simulink model "robot_arm"  (Simulink 7.2)
settings: Solver=ode45  StartTime=0.0  StopTime=inf  RelTol=1e-3
libraries: mblibv1 x31, simulink x4, vrlib x1
settings Model: Creator=eniso  LastModifiedBy=houssein01
settings OptimizationCC: InitFltsAndDblsToZero=on
settings DebuggingCC: SaveWithParameterizedLinksMsg=none
settings GRTTargetCC: TargetFcnLib=ansi_tfl_tmw.mat

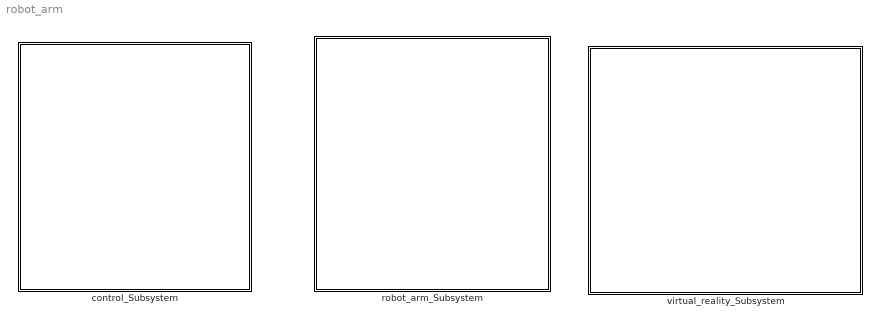
== system robot_arm ==
  control_Subsystem : Subsystem  Orientation=left
  robot_arm_Subsystem : Subsystem
  virtual_reality_Subsystem : Subsystem

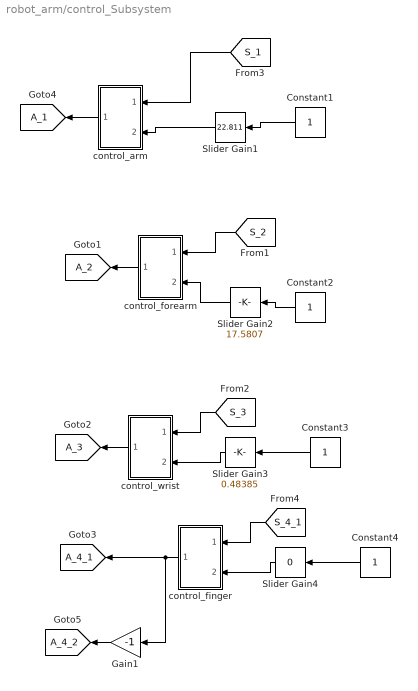
== system robot_arm/control_Subsystem ==
  Constant{1..4} (4 alike) : Constant  Orientation=left  OutDataType=sfix(16)  OutScaling=2^0
  Gain1 : Gain  Orientation=left  Gain=-1  ParameterDataType=sfix(16)  ParameterScaling=2^0  OutDataType=sfix(16)  OutScaling=2^0
  Slider Gain1 : simulink/Math Operations/Slider Gain  Orientation=left  SystemSampleTime=-1  low=-90  gain=22.811  high=90
  Slider Gain2 : simulink/Math Operations/Slider Gain  Orientation=left  SystemSampleTime=-1  low=-25  gain=17.5807  high=30
  Slider Gain3 : simulink/Math Operations/Slider Gain  Orientation=left  SystemSampleTime=-1  low=-25  gain=0.48385  high=45
  Slider Gain4 : simulink/Math Operations/Slider Gain  Orientation=left  SystemSampleTime=-1  low=-10  gain=0  high=0
  control_arm : Subsystem  Orientation=left
  control_finger : Subsystem  Orientation=left
  control_forearm : Subsystem  Orientation=left
  control_wrist : Subsystem  Orientation=left
  tag scope: A_1=global, A_2=global, A_3=global, A_4_1=global, A_4_2=global
  wires:
  Constant1/1 -> Slider Gain1/1
  Slider Gain1/1 -> control_arm/2(In2)
  Constant2/1 -> Slider Gain2/1
  Slider Gain2/1 -> control_forearm/2(In2)
  Constant3/1 -> Slider Gain3/1
  Slider Gain3/1 -> control_wrist/2(In2)
  control_arm/1(Out1) -> [A_1]
  [S_1] -> control_arm/1(In1)
  [S_2] -> control_forearm/1(In1)
  [S_3] -> control_wrist/1(In1)
  control_forearm/1(Out1) -> [A_2]
  control_wrist/1(Out1) -> [A_3]
  Constant4/1 -> Slider Gain4/1
  Slider Gain4/1 -> control_finger/2(In2)
  [S_4_1] -> control_finger/1(In1)
  control_finger/1(Out1) -> [A_4_1], Gain1/1
  Gain1/1 -> [A_4_2]

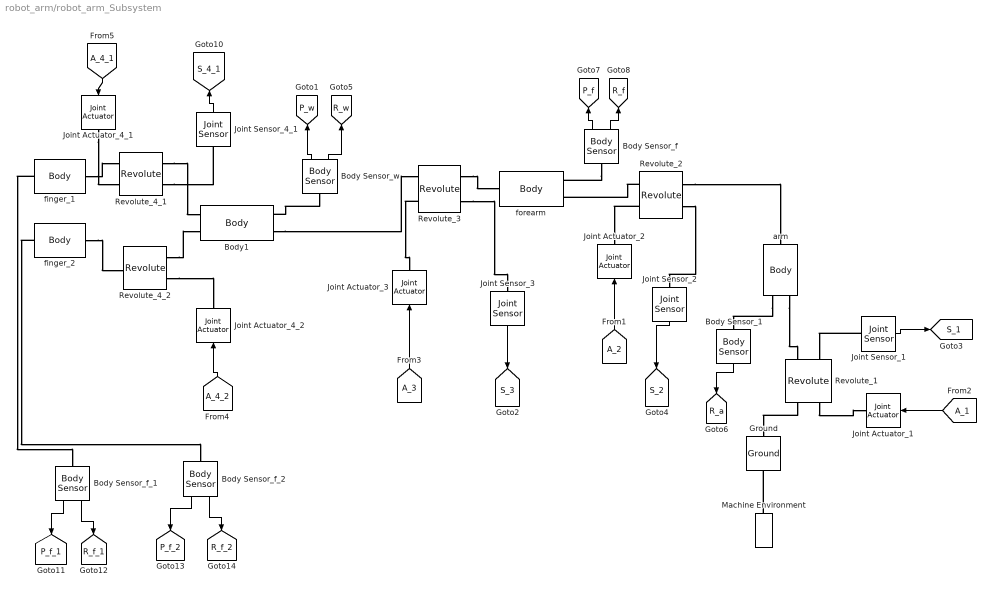
== system robot_arm/robot_arm_Subsystem ==
  Body Sensor_1 : mblibv1/Sensors &  Actuators/Body Sensor  Orientation=down  DialogController=MECH.DynMechDlgSource  SystemSampleTime=-1  UpdateFromCAD=off  PhysicalDomain=Mechanical  PortType=blob  Muxed=off  Pose=on  Angle=on  AngleUnits=deg  ArcVelocity=off  ArcVelocityUnits=deg/s  ArcAcceleration=off  ArcAccelerationUnits=deg/s^2  CoordPosition=off  CoordPositionUnits=m  Velocity=off  VelocityUnits=m/s  Acceleration=off  AccelerationUnits=m/s^2  Quaternion=on  QuaternionDT=off  QuaternionDDT=off  QuaternionUnits=off  OutputVector=[1]  ActiveIO=on  Width=9  DialogClass=MechanicalSensorBlock  ReferenceFrame=Absolute (World)
  Body Sensor_f : mblibv1/Sensors &  Actuators/Body Sensor  Orientation=up  DialogController=MECH.DynMechDlgSource  SystemSampleTime=-1  UpdateFromCAD=off  PhysicalDomain=Mechanical  PortType=blob  Muxed=off  Pose=on  Angle=on  AngleUnits=deg  ArcVelocity=off  ArcVelocityUnits=deg/s  ArcAcceleration=off  ArcAccelerationUnits=deg/s^2  CoordPosition=on  CoordPositionUnits=m  Velocity=off  VelocityUnits=m/s  Acceleration=off  AccelerationUnits=m/s^2  Quaternion=on  QuaternionDT=off  QuaternionDDT=off  QuaternionUnits=off  OutputVector=[1]  ActiveIO=on  Width=12  DialogClass=MechanicalSensorBlock  ReferenceFrame=Absolute (World)
  Body Sensor_f_1 : mblibv1/Sensors &  Actuators/Body Sensor  Orientation=down  DialogController=MECH.DynMechDlgSource  SystemSampleTime=-1  UpdateFromCAD=off  PhysicalDomain=Mechanical  PortType=blob  Muxed=off  Pose=on  Angle=on  AngleUnits=deg  ArcVelocity=off  ArcVelocityUnits=deg/s  ArcAcceleration=off  ArcAccelerationUnits=deg/s^2  CoordPosition=on  CoordPositionUnits=m  Velocity=off  VelocityUnits=m/s  Acceleration=off  AccelerationUnits=m/s^2  Quaternion=on  QuaternionDT=off  QuaternionDDT=off  QuaternionUnits=off  OutputVector=[1]  ActiveIO=on  Width=12  DialogClass=MechanicalSensorBlock  ReferenceFrame=Absolute (World)
  Body Sensor_f_2 : mblibv1/Sensors &  Actuators/Body Sensor  Orientation=down  DialogController=MECH.DynMechDlgSource  SystemSampleTime=-1  UpdateFromCAD=off  PhysicalDomain=Mechanical  PortType=blob  Muxed=off  Pose=on  Angle=on  AngleUnits=deg  ArcVelocity=off  ArcVelocityUnits=deg/s  ArcAcceleration=off  ArcAccelerationUnits=deg/s^2  CoordPosition=on  CoordPositionUnits=m  Velocity=off  VelocityUnits=m/s  Acceleration=off  AccelerationUnits=m/s^2  Quaternion=on  QuaternionDT=off  QuaternionDDT=off  QuaternionUnits=off  OutputVector=[1]  ActiveIO=on  Width=12  DialogClass=MechanicalSensorBlock  ReferenceFrame=Absolute (World)
  Body Sensor_w : mblibv1/Sensors &  Actuators/Body Sensor  Orientation=up  DialogController=MECH.DynMechDlgSource  SystemSampleTime=-1  UpdateFromCAD=off  PhysicalDomain=Mechanical  PortType=blob  Muxed=off  Pose=on  Angle=on  AngleUnits=deg  ArcVelocity=off  ArcVelocityUnits=deg/s  ArcAcceleration=off  ArcAccelerationUnits=deg/s^2  CoordPosition=on  CoordPositionUnits=m  Velocity=off  VelocityUnits=m/s  Acceleration=off  AccelerationUnits=m/s^2  Quaternion=on  QuaternionDT=off  QuaternionDDT=off  QuaternionUnits=off  OutputVector=[1]  ActiveIO=on  Width=12  DialogClass=MechanicalSensorBlock  ReferenceFrame=Absolute (World)
  Body1 : mblibv1/Bodies/Body  Orientation=left  DialogController=MECH.DynMechDlgSource  PhysicalDomain=mechanical  SubClassName=Unknown  LeftPortType=workingframe  RightPortType=workingframe  LConnTagsString=CG|CS1  RConnTagsString=CS3|CS2  UpdateFromCAD=off  DialogClass=MechanicalBodyBlock  Mass=1.9  MassUnits=kg  InertiaUnits=kg*m^2  Inertia=[0.0038 0 0 ; 0 0.0005 0 ;0 0 0.0038]  Shape=Cylinder  ShapeDims=[1 1]  ShapeUnits=m  ShapeUse=false  Density=1  DensityUnits=kg/m^3  DensityUse=false  GraphicsMode=MACHINE_DEFAULT  BodyColorSelMode=MACHINE_DEFAULT  BodyColor=[1 0 0]  AttachedToCS=CG  CG=Left$CG$[0 0.1 0]$CS1$CS1$m$[0 0 0]$Euler X-Y-Z$deg$CS1$true$none  WorkingFrames=Right$CS3$[0 0.2 0.03]$CS1$CS1$m$[0 0 0]$Euler X-Y-Z$deg$CS1$true$none#Left$CS1$[0 0 0]$World$Adjoining$m$[0 0 45]$Euler X-Y-Z$deg$Adjoining$true$none#Right$CS2$[0 0.2 -0.03]$CS1$CS1$m$[0 0 0]$Euler X-Y-Z$deg$CS1$true$none  CGPos=[0 0.1 0]  CGRot=[0 0 0]  CS0Pos=[]  CS0Rot=[]  CS1Pos=[0 0 0]  CS1Rot=[0 0 45]  CS2Pos=[0 0.2 -0.03]  CS2Rot=[0 0 0]  CS3Pos=[0 0.2 0.03]  CS3Rot=[0 0 0]  CS4Pos=[]  CS4Rot=[]  CS5Pos=[]  CS5Rot=[]  CS6Pos=[]  CS6Rot=[]  CS7Pos=[]  CS7Rot=[]  CS8Pos=[]  CS8Rot=[]  CS9Pos=[]  CS9Rot=[]  CS10Pos=[]  CS10Rot=[]  CS11Pos=[]  CS11Rot=[]  CS12Pos=[]  CS12Rot=[]  CS13Pos=[]  CS13Rot=[]  CS14Pos=[]  CS14Rot=[]  CS15Pos=[]  CS15Rot=[]  CS16Pos=[]  CS16Rot=[]  CS17Pos=[]  CS17Rot=[]  CS18Pos=[]  CS18Rot=[]  CS19Pos=[]  CS19Rot=[]  CS20Pos=[]  CS20Rot=[]
  Ground : mblibv1/Bodies/Ground  Orientation=up  DialogController=MECH.DynMechDlgSource  SystemSampleTime=-1  UpdateFromCAD=off  LeftPortType=env  RightPortType=workingframe  PhysicalDomain=Mechanical  DialogClass=GroundBlock  CoordPosition=[0 0 0]  CoordPositionUnits=m  StateVectorMgrId=1  MachineId=[2 0]  ShowEnvPort=on
  Joint Actuator_1 : mblibv1/Sensors &  Actuators/Joint Actuator  Orientation=left  DialogController=MECH.DynMechDlgSource  SystemSampleTime=-1  UpdateFromCAD=off  PhysicalDomain=Mechanical  PortType=blob  ActuationStyle=Motion  AngleUnits=deg  ArcVelocityUnits=deg/s  ArcAccelerationUnits=deg/s^2  CoordPositionUnits=m  VelocityUnits=m/s  AccelerationUnits=m/s^2  ForceUnits=N  TorqueUnits=N*m  ActiveIO=on  Width=3  DialogClass=MechanicalActuatorBlock  Primitive=R1  ReferenceFrame=Absolute (INERTIAL)
  Joint Actuator_2 : mblibv1/Sensors &  Actuators/Joint Actuator  Orientation=up  DialogController=MECH.DynMechDlgSource  SystemSampleTime=-1  UpdateFromCAD=off  PhysicalDomain=Mechanical  PortType=blob  ActuationStyle=Motion  AngleUnits=deg  ArcVelocityUnits=deg/s  ArcAccelerationUnits=deg/s^2  CoordPositionUnits=m  VelocityUnits=m/s  AccelerationUnits=m/s^2  ForceUnits=N  TorqueUnits=N*m  ActiveIO=on  Width=3  DialogClass=MechanicalActuatorBlock  Primitive=R1  ReferenceFrame=Absolute (INERTIAL)
  Joint Actuator_3 : mblibv1/Sensors &  Actuators/Joint Actuator  Orientation=up  DialogController=MECH.DynMechDlgSource  SystemSampleTime=-1  UpdateFromCAD=off  PhysicalDomain=Mechanical  PortType=blob  ActuationStyle=Motion  AngleUnits=deg  ArcVelocityUnits=deg/s  ArcAccelerationUnits=deg/s^2  CoordPositionUnits=m  VelocityUnits=m/s  AccelerationUnits=m/s^2  ForceUnits=N  TorqueUnits=N*m  ActiveIO=on  Width=3  DialogClass=MechanicalActuatorBlock  Primitive=R1  ReferenceFrame=Absolute (INERTIAL)
  Joint Actuator_4_1 : mblibv1/Sensors &  Actuators/Joint Actuator  Orientation=down  DialogController=MECH.DynMechDlgSource  SystemSampleTime=-1  UpdateFromCAD=off  PhysicalDomain=Mechanical  PortType=blob  ActuationStyle=Motion  AngleUnits=deg  ArcVelocityUnits=deg/s  ArcAccelerationUnits=deg/s^2  CoordPositionUnits=m  VelocityUnits=m/s  AccelerationUnits=m/s^2  ForceUnits=N  TorqueUnits=N*m  ActiveIO=on  Width=3  DialogClass=MechanicalActuatorBlock  Primitive=R1  ReferenceFrame=Absolute (INERTIAL)
  Joint Actuator_4_2 : mblibv1/Sensors &  Actuators/Joint Actuator  Orientation=up  DialogController=MECH.DynMechDlgSource  SystemSampleTime=-1  UpdateFromCAD=off  PhysicalDomain=Mechanical  PortType=blob  ActuationStyle=Motion  AngleUnits=deg  ArcVelocityUnits=deg/s  ArcAccelerationUnits=deg/s^2  CoordPositionUnits=m  VelocityUnits=m/s  AccelerationUnits=m/s^2  ForceUnits=N  TorqueUnits=N*m  ActiveIO=on  Width=3  DialogClass=MechanicalActuatorBlock  Primitive=R1  ReferenceFrame=Absolute (INERTIAL)
  Joint Sensor_1 : mblibv1/Sensors &  Actuators/Joint Sensor  DialogController=MECH.DynMechDlgSource  SystemSampleTime=-1  UpdateFromCAD=off  PhysicalDomain=Mechanical  PortType=blob  Muxed=on  Pose=off  Angle=on  AngleUnits=deg  ArcVelocity=off  ArcVelocityUnits=deg/s  ArcAcceleration=off  ArcAccelerationUnits=deg/s^2  CoordPosition=on  CoordPositionUnits=m  Velocity=off  VelocityUnits=m/s  Acceleration=off  AccelerationUnits=m/s^2  Quaternion=on  QuaternionDT=off  QuaternionDDT=off  QuaternionUnits=off  OutputVector=[1]  ActiveIO=on  Width=1  DialogClass=MechanicalSensorBlock  Primitive=R1  Force=off  ForceUnits=N  Torque=off  TorqueUnits=N*m  ReferenceFrame=Absolute (World)  ReactionSensedSide=Base  ReactionReferenceFrame=Absolute (World)  ReactionForce=off  ReactionForceUnits=N  ReactionMoment=off  ReactionMomentUnits=N*m
  Joint Sensor_2 : mblibv1/Sensors &  Actuators/Joint Sensor  Orientation=down  DialogController=MECH.DynMechDlgSource  SystemSampleTime=-1  UpdateFromCAD=off  PhysicalDomain=Mechanical  PortType=blob  Muxed=on  Pose=off  Angle=on  AngleUnits=deg  ArcVelocity=off  ArcVelocityUnits=deg/s  ArcAcceleration=off  ArcAccelerationUnits=deg/s^2  CoordPosition=on  CoordPositionUnits=m  Velocity=off  VelocityUnits=m/s  Acceleration=off  AccelerationUnits=m/s^2  Quaternion=on  QuaternionDT=off  QuaternionDDT=off  QuaternionUnits=off  OutputVector=[1]  ActiveIO=on  Width=1  DialogClass=MechanicalSensorBlock  Primitive=R1  Force=off  ForceUnits=N  Torque=off  TorqueUnits=N*m  ReferenceFrame=Absolute (World)  ReactionSensedSide=Base  ReactionReferenceFrame=Absolute (World)  ReactionForce=off  ReactionForceUnits=N  ReactionMoment=off  ReactionMomentUnits=N*m
  Joint Sensor_3 : mblibv1/Sensors &  Actuators/Joint Sensor  Orientation=down  DialogController=MECH.DynMechDlgSource  SystemSampleTime=-1  UpdateFromCAD=off  PhysicalDomain=Mechanical  PortType=blob  Muxed=on  Pose=off  Angle=on  AngleUnits=deg  ArcVelocity=off  ArcVelocityUnits=deg/s  ArcAcceleration=off  ArcAccelerationUnits=deg/s^2  CoordPosition=on  CoordPositionUnits=m  Velocity=off  VelocityUnits=m/s  Acceleration=off  AccelerationUnits=m/s^2  Quaternion=on  QuaternionDT=off  QuaternionDDT=off  QuaternionUnits=off  OutputVector=[1]  ActiveIO=on  Width=1  DialogClass=MechanicalSensorBlock  Primitive=R1  Force=off  ForceUnits=N  Torque=off  TorqueUnits=N*m  ReferenceFrame=Absolute (World)  ReactionSensedSide=Base  ReactionReferenceFrame=Absolute (World)  ReactionForce=off  ReactionForceUnits=N  ReactionMoment=off  ReactionMomentUnits=N*m
  Joint Sensor_4_1 : mblibv1/Sensors &  Actuators/Joint Sensor  Orientation=up  DialogController=MECH.DynMechDlgSource  SystemSampleTime=-1  UpdateFromCAD=off  PhysicalDomain=Mechanical  PortType=blob  Muxed=on  Pose=off  Angle=on  AngleUnits=deg  ArcVelocity=off  ArcVelocityUnits=deg/s  ArcAcceleration=off  ArcAccelerationUnits=deg/s^2  CoordPosition=on  CoordPositionUnits=m  Velocity=off  VelocityUnits=m/s  Acceleration=off  AccelerationUnits=m/s^2  Quaternion=on  QuaternionDT=off  QuaternionDDT=off  QuaternionUnits=off  OutputVector=[1]  ActiveIO=on  Width=1  DialogClass=MechanicalSensorBlock  Primitive=R1  Force=off  ForceUnits=N  Torque=off  TorqueUnits=N*m  ReferenceFrame=Absolute (World)  ReactionSensedSide=Base  ReactionReferenceFrame=Absolute (World)  ReactionForce=off  ReactionForceUnits=N  ReactionMoment=off  ReactionMomentUnits=N*m
  Machine Environment : mblibv1/Bodies/Machine Environment  Orientation=up  DialogController=MECH.DialogSource  SystemSampleTime=-1  PortType=env  PhysicalDomain=Mechanical  DialogTemplateClass=MECH.MachineEnvironment  SyncWhenCopied=off  Gravity="[0  0 -9.81]"  GravityUnits=m/s^2  GravityAsSignal=off  Dimensionality=Auto-detect  AnalysisType=Forward dynamics  LinearAssemblyTolerance=1e-3  LinearAssemblyToleranceUnits=m  AngularAssemblyTolerance=1e-3  AngularAssemblyToleranceUnits=deg  ConstraintSolverType=Stabilizing  ConstraintRelTolerance=1e-4  ConstraintAbsTolerance=1e-4  UseRobustSingularityHandling=off  RedundancyAnalysisToleranceType=Automatically select tolerance  RedundancyAnalysisTolerance=1e-14  StatePerturbationType=Fixed  PerturbationSize=1e-5  VisualizeMachine=on  BodyVisualizationType=Use model default body geometries  BodyColorSelMode=Use model default  DefaultBodyColor=[1 0 0]
  Revolute_1 : mblibv1/Joints/Revolute  Orientation=up  DialogController=MECH.DynMechDlgSource  PhysicalDomain=mechanical  SubClassName=Unknown  LeftPortType=blob  RightPortType=blob  LConnTagsString=__newl0|SA1  RConnTagsString=__newr0|SA1  UpdateFromCAD=off  NumSAPorts=2  CutJoint=off  MarkAsCut=off  Primitives=prismatic  PrimitiveProps=R1$World$[0 1 0]$revolute  DialogClass=JointBlock  R1Axis=[0 1 0]
  Revolute_2 : mblibv1/Joints/Revolute  Orientation=left  DialogController=MECH.DynMechDlgSource  PhysicalDomain=mechanical  SubClassName=Unknown  LeftPortType=blob  RightPortType=blob  LConnTagsString=__newl0|SA1  RConnTagsString=__newr0|SA1  UpdateFromCAD=off  NumSAPorts=2  CutJoint=off  MarkAsCut=off  Primitives=prismatic  PrimitiveProps=R1$Base$[ 0 0 1]$revolute  DialogClass=JointBlock  R1Axis=[ 0 0 1]
  Revolute_3 : mblibv1/Joints/Revolute  Orientation=left  DialogController=MECH.DynMechDlgSource  PhysicalDomain=mechanical  SubClassName=Unknown  LeftPortType=blob  RightPortType=blob  LConnTagsString=__newl0|SA1  RConnTagsString=__newr0|SA1  UpdateFromCAD=off  NumSAPorts=2  CutJoint=off  MarkAsCut=off  Primitives=prismatic  PrimitiveProps=R1$Base$[0 0 1 ]$revolute  DialogClass=JointBlock  R1Axis=[0 0 1 ]
  Revolute_4_1 : mblibv1/Joints/Revolute  Orientation=left  DialogController=MECH.DynMechDlgSource  PhysicalDomain=mechanical  SubClassName=Unknown  LeftPortType=blob  RightPortType=blob  LConnTagsString=__newl0|SA1  RConnTagsString=__newr0|SA1  UpdateFromCAD=off  NumSAPorts=2  CutJoint=off  MarkAsCut=off  Primitives=prismatic  PrimitiveProps="R1$Base$[1 0  0 ]$revolute"  DialogClass=JointBlock  R1Axis="[1 0  0 ]"
  Revolute_4_2 : mblibv1/Joints/Revolute  Orientation=left  DialogController=MECH.DynMechDlgSource  PhysicalDomain=mechanical  SubClassName=Unknown  LeftPortType=blob  RightPortType=blob  LConnTagsString=__newl0|SA1  RConnTagsString=__newr0  UpdateFromCAD=off  NumSAPorts=1  CutJoint=off  MarkAsCut=off  Primitives=prismatic  PrimitiveProps=R1$Base$[1 0 0 ]$revolute  DialogClass=JointBlock  R1Axis=[1 0 0 ]
  arm : mblibv1/Bodies/Body  Orientation=up  DialogController=MECH.DynMechDlgSource  PhysicalDomain=mechanical  SubClassName=Unknown  LeftPortType=workingframe  RightPortType=workingframe  LConnTagsString=CG|CS1  RConnTagsString=CS4  UpdateFromCAD=off  DialogClass=MechanicalBodyBlock  Mass=15.86  MassUnits=kg  InertiaUnits=kg*m^2  Inertia=[0.066 0 0 ; 0 0.026 0 ; 0 0 0.066]  Shape=Cylinder  ShapeDims=[1 1]  ShapeUnits=m  ShapeUse=false  Density=1  DensityUnits=kg/m^3  DensityUse=false  GraphicsMode=MACHINE_DEFAULT  BodyColorSelMode=MACHINE_DEFAULT  BodyColor=[1 0 0]  AttachedToCS=CG  CG="Left$CG$[0  0.1 0]$World$CS1$m$[0 0 0]$Euler X-Y-Z$deg$WORLD$true$none"  WorkingFrames="Left$CS1$[0 0 0]$World$Adjoining$m$[0 0 0]$Euler X-Y-Z$deg$WORLD$true$none#Right$CS2$[0  0.2 0]$World$CS1$m$[0 0 0]$Euler X-Y-Z$deg$WORLD$false$none#Right$CS4$[0  0.16 0]$World$CS1$m$[0 0 0]$Euler X-Y-Z$deg$WORLD$true$none"  CGPos="[0  0.1 0]"  CGRot=[0 0 0]  CS0Pos=[]  CS0Rot=[]  CS1Pos=[0 0 0]  CS1Rot=[0 0 0]  CS2Pos="[0  0.2 0]"  CS2Rot=[0 0 0]  CS3Pos=[]  CS3Rot=[]  CS4Pos="[0  0.16 0]"  CS4Rot=[0 0 0]  CS5Pos=[]  CS5Rot=[]  CS6Pos=[]  CS6Rot=[]  CS7Pos=[]  CS7Rot=[]  CS8Pos=[]  CS8Rot=[]  CS9Pos=[]  CS9Rot=[]  CS10Pos=[]  CS10Rot=[]  CS11Pos=[]  CS11Rot=[]  CS12Pos=[]  CS12Rot=[]  CS13Pos=[]  CS13Rot=[]  CS14Pos=[]  CS14Rot=[]  CS15Pos=[]  CS15Rot=[]  CS16Pos=[]  CS16Rot=[]  CS17Pos=[]  CS17Rot=[]  CS18Pos=[]  CS18Rot=[]  CS19Pos=[]  CS19Rot=[]  CS20Pos=[]  CS20Rot=[]
  finger_1 : mblibv1/Bodies/Body  Orientation=left  DialogController=MECH.DynMechDlgSource  PhysicalDomain=mechanical  SubClassName=Unknown  LeftPortType=workingframe  RightPortType=workingframe  LConnTagsString=CS1  RConnTagsString=CG  UpdateFromCAD=off  DialogClass=MechanicalBodyBlock  Mass=0.158  MassUnits=kg  InertiaUnits=kg*m^2  Inertia=[0.000038 0 0 ; 0 0.00001050 0 ; 0 0 0.000038]  Shape=Cylinder  ShapeDims=[1 1]  ShapeUnits=m  ShapeUse=false  Density=1  DensityUnits=kg/m^3  DensityUse=false  GraphicsMode=MACHINE_DEFAULT  BodyColorSelMode=MACHINE_DEFAULT  BodyColor=[1 0 0]  AttachedToCS=CG  CG=Right$CG$[ 0 0.03 0 ]$CS1$CS1$m$[0 0 0]$Euler X-Y-Z$deg$CS1$true$none  WorkingFrames="Left$CS1$[0 0 0]$Adjoining$Adjoining$m$[0 0 0]$Euler X-Y-Z$deg$Adjoining$true$none#Right$CS2$[0 0.06 0  ]$CS1$CS1$m$[0 0 0]$Euler X-Y-Z$deg$CS1$false$none"  CGPos=[ 0 0.03 0 ]  CGRot=[0 0 0]  CS0Pos=[]  CS0Rot=[]  CS1Pos=[0 0 0]  CS1Rot=[0 0 0]  CS2Pos="[0 0.06 0  ]"  CS2Rot=[0 0 0]  CS3Pos=[]  CS3Rot=[]  CS4Pos=[]  CS4Rot=[]  CS5Pos=[]  CS5Rot=[]  CS6Pos=[]  CS6Rot=[]  CS7Pos=[]  CS7Rot=[]  CS8Pos=[]  CS8Rot=[]  CS9Pos=[]  CS9Rot=[]  CS10Pos=[]  CS10Rot=[]  CS11Pos=[]  CS11Rot=[]  CS12Pos=[]  CS12Rot=[]  CS13Pos=[]  CS13Rot=[]  CS14Pos=[]  CS14Rot=[]  CS15Pos=[]  CS15Rot=[]  CS16Pos=[]  CS16Rot=[]  CS17Pos=[]  CS17Rot=[]  CS18Pos=[]  CS18Rot=[]  CS19Pos=[]  CS19Rot=[]  CS20Pos=[]  CS20Rot=[]
  finger_2 : mblibv1/Bodies/Body  Orientation=left  DialogController=MECH.DynMechDlgSource  PhysicalDomain=mechanical  SubClassName=Unknown  LeftPortType=workingframe  RightPortType=workingframe  LConnTagsString=CS1  RConnTagsString=CG  UpdateFromCAD=off  DialogClass=MechanicalBodyBlock  Mass=0.158  MassUnits=kg  InertiaUnits=kg*m^2  Inertia=[0.000038 0 0 ; 0 0.00001050 0 ; 0 0 0.000038]  Shape=Cylinder  ShapeDims=[1 1]  ShapeUnits=m  ShapeUse=false  Density=1  DensityUnits=kg/m^3  DensityUse=false  GraphicsMode=MACHINE_DEFAULT  BodyColorSelMode=MACHINE_DEFAULT  BodyColor=[1 0 0]  AttachedToCS=CG  CG=Right$CG$[0 0.03 0 ]$CS1$CS1$m$[0 0 0]$Euler X-Y-Z$deg$CS1$true$none  WorkingFrames=Left$CS1$[0 0 0]$Adjoining$Adjoining$m$[0 0 0]$Euler X-Y-Z$deg$Adjoining$true$none#Right$CS2$[0 0.06 0 ]$CS1$CS1$m$[0 0 0]$Euler X-Y-Z$deg$CS1$false$none  CGPos=[0 0.03 0 ]  CGRot=[0 0 0]  CS0Pos=[]  CS0Rot=[]  CS1Pos=[0 0 0]  CS1Rot=[0 0 0]  CS2Pos=[0 0.06 0 ]  CS2Rot=[0 0 0]  CS3Pos=[]  CS3Rot=[]  CS4Pos=[]  CS4Rot=[]  CS5Pos=[]  CS5Rot=[]  CS6Pos=[]  CS6Rot=[]  CS7Pos=[]  CS7Rot=[]  CS8Pos=[]  CS8Rot=[]  CS9Pos=[]  CS9Rot=[]  CS10Pos=[]  CS10Rot=[]  CS11Pos=[]  CS11Rot=[]  CS12Pos=[]  CS12Rot=[]  CS13Pos=[]  CS13Rot=[]  CS14Pos=[]  CS14Rot=[]  CS15Pos=[]  CS15Rot=[]  CS16Pos=[]  CS16Rot=[]  CS17Pos=[]  CS17Rot=[]  CS18Pos=[]  CS18Rot=[]  CS19Pos=[]  CS19Rot=[]  CS20Pos=[]  CS20Rot=[]
  forearm : mblibv1/Bodies/Body  Orientation=left  DialogController=MECH.DynMechDlgSource  PhysicalDomain=mechanical  SubClassName=Unknown  LeftPortType=workingframe  RightPortType=workingframe  LConnTagsString=CG|CS1  RConnTagsString=CS2  UpdateFromCAD=off  DialogClass=MechanicalBodyBlock  Mass=4.758  MassUnits=kg  InertiaUnits=kg*m^2  Inertia=[0.0254 0 0 ; 0 0.00206 0; 0 0 0.0262]  Shape=Cylinder  ShapeDims=[1 1]  ShapeUnits=m  ShapeUse=false  Density=1  DensityUnits=kg/m^3  DensityUse=false  GraphicsMode=MACHINE_DEFAULT  BodyColorSelMode=MACHINE_DEFAULT  BodyColor=[1 0 0]  AttachedToCS=CG  CG=Left$CG$[0 0.15 0]$CS1$CS1$m$[0 0 0]$Euler X-Y-Z$deg$CS1$true$none  WorkingFrames="Left$CS1$[0 0 0]$World$Adjoining$m$[0 0 45]$Euler X-Y-Z$deg$World$true$none#Left$CS4$[0 0 0]$CS1$CS1$m$[0 0 0]$Euler X-Y-Z$deg$CS1$false$none#Right$CS2$[0  0.3 0]$CS1$CS1$m$[0 0 0]$Euler X-Y-Z$deg$CS1$true$none"  CGPos=[0 0.15 0]  CGRot=[0 0 0]  CS0Pos=[]  CS0Rot=[]  CS1Pos=[0 0 0]  CS1Rot=[0 0 45]  CS2Pos="[0  0.3 0]"  CS2Rot=[0 0 0]  CS3Pos=[]  CS3Rot=[]  CS4Pos=[0 0 0]  CS4Rot=[0 0 0]  CS5Pos=[]  CS5Rot=[]  CS6Pos=[]  CS6Rot=[]  CS7Pos=[]  CS7Rot=[]  CS8Pos=[]  CS8Rot=[]  CS9Pos=[]  CS9Rot=[]  CS10Pos=[]  CS10Rot=[]  CS11Pos=[]  CS11Rot=[]  CS12Pos=[]  CS12Rot=[]  CS13Pos=[]  CS13Rot=[]  CS14Pos=[]  CS14Rot=[]  CS15Pos=[]  CS15Rot=[]  CS16Pos=[]  CS16Rot=[]  CS17Pos=[]  CS17Rot=[]  CS18Pos=[]  CS18Rot=[]  CS19Pos=[]  CS19Rot=[]  CS20Pos=[]  CS20Rot=[]
  tag scope: P_f=global, P_f_1=global, P_f_2=global, P_w=global, R_a=global, R_f=global, R_f_1=global, R_f_2=global, R_w=global, S_1=global, S_2=global, S_3=global, S_4_1=global
  wires:
  Joint Sensor_3/1 -> [S_3]
  Joint Sensor_1/1 -> [S_1]
  Joint Sensor_2/1 -> [S_2]
  [A_3] -> Joint Actuator_3/1
  [A_2] -> Joint Actuator_2/1
  Body Sensor_1/1 -> [R_a]
  Body Sensor_f/1 -> [P_f]
  Body Sensor_f/2 -> [R_f]
  Body Sensor_w/2 -> [R_w]
  Body Sensor_w/1 -> [P_w]
  [A_4_2] -> Joint Actuator_4_2/1
  Joint Sensor_4_1/1 -> [S_4_1]
  [A_4_1] -> Joint Actuator_4_1/1
  [A_1] -> Joint Actuator_1/1
  Body Sensor_f_1/2 -> [R_f_1]
  Body Sensor_f_1/1 -> [P_f_1]
  Body Sensor_f_2/2 -> [R_f_2]
  Body Sensor_f_2/1 -> [P_f_2]
  connections:
  arm/LConn1 -- Body Sensor_1/LConn1
  Body Sensor_f/LConn1 -- forearm/LConn1
  finger_1/RConn1 -- Body Sensor_f_1/LConn1
  finger_2/RConn1 -- Body Sensor_f_2/LConn1
  Body Sensor_w/LConn1 -- Body1/LConn1
  Body1/LConn2 -- Revolute_3/RConn1
  Revolute_4_1/LConn1 -- Body1/RConn1
  Revolute_4_2/LConn1 -- Body1/RConn2
  Machine Environment/RConn1 -- Ground/LConn1
  Revolute_1/LConn1 -- Ground/RConn1
  Revolute_1/LConn2 -- Joint Actuator_1/RConn1
  Revolute_2/RConn2 -- Joint Actuator_2/RConn1
  Revolute_3/RConn2 -- Joint Actuator_3/RConn1
  Joint Actuator_4_1/RConn1 -- Revolute_4_1/RConn2
  Revolute_4_2/LConn2 -- Joint Actuator_4_2/RConn1
  Joint Sensor_1/LConn1 -- Revolute_1/RConn2
  Revolute_2/LConn2 -- Joint Sensor_2/LConn1
  Revolute_3/LConn2 -- Joint Sensor_3/LConn1
  Revolute_4_1/LConn2 -- Joint Sensor_4_1/LConn1
  arm/LConn2 -- Revolute_1/RConn1
  Revolute_2/LConn1 -- arm/RConn1
  Revolute_2/RConn1 -- forearm/LConn2
  Revolute_3/LConn1 -- forearm/RConn1
  finger_1/LConn1 -- Revolute_4_1/RConn1
  finger_2/LConn1 -- Revolute_4_2/RConn1

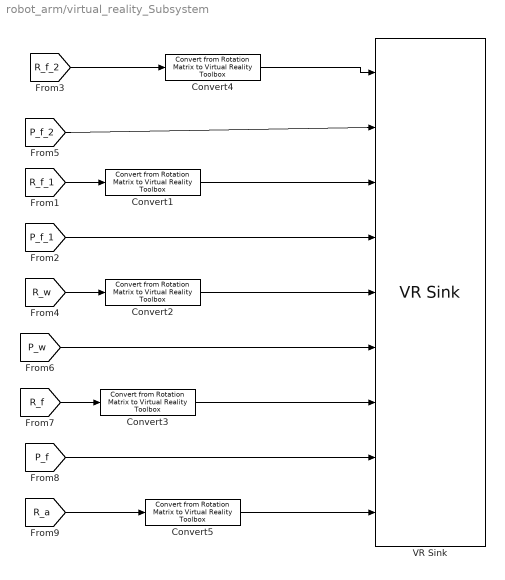
== system robot_arm/virtual_reality_Subsystem ==
  Convert{1..5} (5 alike) : mblibv1/Utilities/Convert from Rotation Matrix to Virtual Reality Toolbox  Tag=Pose2VR
  VR Sink : vrlib/VR Sink  SampleTime=0.1  ViewEnable=on  RemoteChange=off  RemoteView=off  FieldsWritten=finger_2.rotation.4.1.double#finger_2.translation.3.1.double#finger_1.rotation.4.1.double#finger_1.translation.3.1.double#wrist.rotation.4.1.double#wrist.translation.3.1.double#forearm.rotation.4.1.double#forearm.translation.3.1.double#arm.rotation.4.1.double  WorldFileName=robot_arm.wrl  WorldDescription=robot_arm-project  AutoView=on  VideoDimensions=[]
  wires:
  [R_f_2] -> Convert4/1
  [R_f_1] -> Convert1/1
  [R_w] -> Convert2/1
  [R_f] -> Convert3/1
  [R_a] -> Convert5/1
  Convert4/1 -> VR Sink/1
  [P_f_2] -> VR Sink/2
  Convert1/1 -> VR Sink/3
  [P_f_1] -> VR Sink/4
  Convert2/1 -> VR Sink/5
  [P_w] -> VR Sink/6
  Convert3/1 -> VR Sink/7
  [P_f] -> VR Sink/8
  Convert5/1 -> VR Sink/9

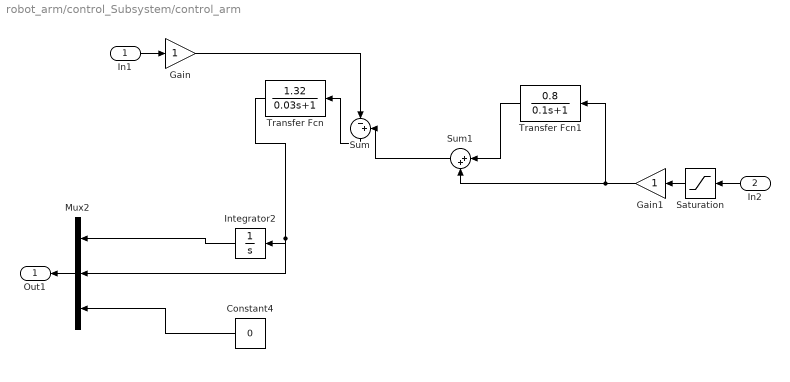
== system robot_arm/control_Subsystem/control_arm ==
  In1 : Inport
  In2 : Inport  Orientation=left  Port=2
  Constant4 : Constant  Orientation=left  Value=0  OutDataType=sfix(16)  OutScaling=2^0
  Gain : Gain  ParameterDataType=sfix(16)  ParameterScaling=2^0  OutDataType=sfix(16)  OutScaling=2^0
  Gain1 : Gain  Orientation=left  ParameterDataType=sfix(16)  ParameterScaling=2^0  OutDataType=sfix(16)  OutScaling=2^0
  Integrator2 : Integrator  Orientation=left
  Mux2 : Mux  Orientation=left  Inputs=3
  Saturation : Saturate  Orientation=left  UpperLimit=90  LowerLimit=-90  OutMin=[-90]  OutMax=[90]  OutDataType=sfix(16)  OutScaling=2^0
  Sum : Sum  Orientation=down  Inputs=|-+  OutDataType=sfix(16)  OutScaling=2^0
  Sum1 : Sum  Orientation=left  Inputs=|++  OutDataType=sfix(16)  OutScaling=2^0
  Transfer Fcn : TransferFcn  Orientation=left  Numerator=[1.32]  Denominator=[0.03 1]
  Transfer Fcn1 : TransferFcn  Orientation=left  Numerator=[0.8]  Denominator=[0.1 1]
  Out1 : Outport  Orientation=left
  wires:
  Sum/1 -> Transfer Fcn/1
  Gain/1 -> Sum/1
  Integrator2/1 -> Mux2/1
  Transfer Fcn/1 -> Integrator2/1, Mux2/2
  Constant4/1 -> Mux2/3
  In1/1 -> Gain/1
  In2/1 -> Saturation/1
  Mux2/1 -> Out1/1
  Sum1/1 -> Sum/2
  Transfer Fcn1/1 -> Sum1/1
  Gain1/1 -> Sum1/2, Transfer Fcn1/1
  Saturation/1 -> Gain1/1

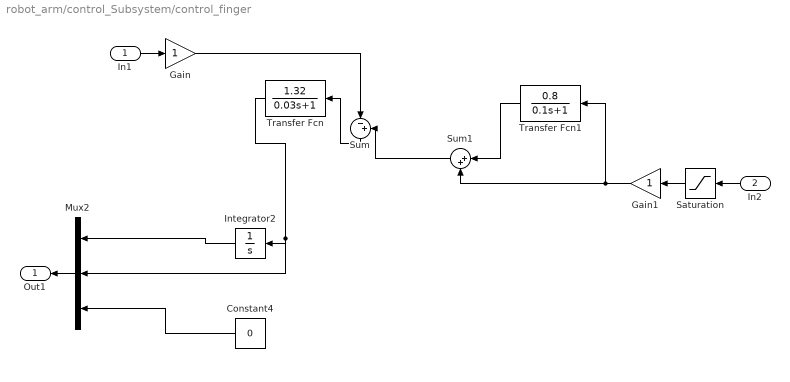
== system robot_arm/control_Subsystem/control_finger ==
  In1 : Inport
  In2 : Inport  Orientation=left  Port=2
  Constant4 : Constant  Orientation=left  Value=0  OutDataType=sfix(16)  OutScaling=2^0
  Gain : Gain  ParameterDataType=sfix(16)  ParameterScaling=2^0  OutDataType=sfix(16)  OutScaling=2^0
  Gain1 : Gain  Orientation=left  ParameterDataType=sfix(16)  ParameterScaling=2^0  OutDataType=sfix(16)  OutScaling=2^0
  Integrator2 : Integrator  Orientation=left
  Mux2 : Mux  Orientation=left  Inputs=3
  Saturation : Saturate  Orientation=left  UpperLimit=80  LowerLimit=-90  OutMin=[-90]  OutMax=[90]  OutDataType=sfix(16)  OutScaling=2^0
  Sum : Sum  Orientation=down  Inputs=|-+  OutDataType=sfix(16)  OutScaling=2^0
  Sum1 : Sum  Orientation=left  Inputs=|++  OutDataType=sfix(16)  OutScaling=2^0
  Transfer Fcn : TransferFcn  Orientation=left  Numerator=[1.32]  Denominator=[0.03 1]
  Transfer Fcn1 : TransferFcn  Orientation=left  Numerator=[0.8]  Denominator=[0.1 1]
  Out1 : Outport  Orientation=left
  wires:
  Sum/1 -> Transfer Fcn/1
  Gain/1 -> Sum/1
  Integrator2/1 -> Mux2/1
  Transfer Fcn/1 -> Integrator2/1, Mux2/2
  Constant4/1 -> Mux2/3
  In1/1 -> Gain/1
  In2/1 -> Saturation/1
  Mux2/1 -> Out1/1
  Sum1/1 -> Sum/2
  Saturation/1 -> Gain1/1
  Gain1/1 -> Transfer Fcn1/1, Sum1/2
  Transfer Fcn1/1 -> Sum1/1

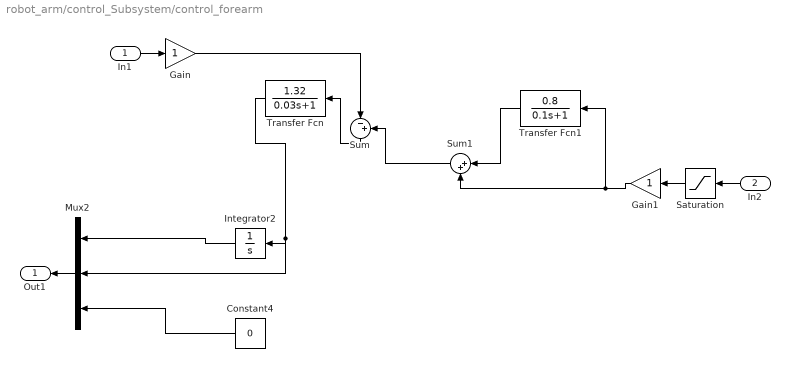
== system robot_arm/control_Subsystem/control_forearm ==
  In1 : Inport
  In2 : Inport  Orientation=left  Port=2
  Constant4 : Constant  Orientation=left  Value=0  OutDataType=sfix(16)  OutScaling=2^0
  Gain : Gain  ParameterDataType=sfix(16)  ParameterScaling=2^0  OutDataType=sfix(16)  OutScaling=2^0
  Gain1 : Gain  Orientation=left  ParameterDataType=sfix(16)  ParameterScaling=2^0  OutDataType=sfix(16)  OutScaling=2^0
  Integrator2 : Integrator  Orientation=left
  Mux2 : Mux  Orientation=left  Inputs=3
  Saturation : Saturate  Orientation=left  UpperLimit=80  LowerLimit=-90  OutMin=[-90]  OutMax=[90]  OutDataType=sfix(16)  OutScaling=2^0
  Sum : Sum  Orientation=down  Inputs=|-+  OutDataType=sfix(16)  OutScaling=2^0
  Sum1 : Sum  Orientation=left  Inputs=|++  OutDataType=sfix(16)  OutScaling=2^0
  Transfer Fcn : TransferFcn  Orientation=left  Numerator=[1.32]  Denominator=[0.03 1]
  Transfer Fcn1 : TransferFcn  Orientation=left  Numerator=[0.8]  Denominator=[0.1 1]
  Out1 : Outport  Orientation=left
  wires:
  Sum/1 -> Transfer Fcn/1
  Gain/1 -> Sum/1
  Integrator2/1 -> Mux2/1
  Transfer Fcn/1 -> Integrator2/1, Mux2/2
  Constant4/1 -> Mux2/3
  In1/1 -> Gain/1
  In2/1 -> Saturation/1
  Mux2/1 -> Out1/1
  Saturation/1 -> Gain1/1
  Sum1/1 -> Sum/2
  Gain1/1 -> Transfer Fcn1/1, Sum1/2
  Transfer Fcn1/1 -> Sum1/1

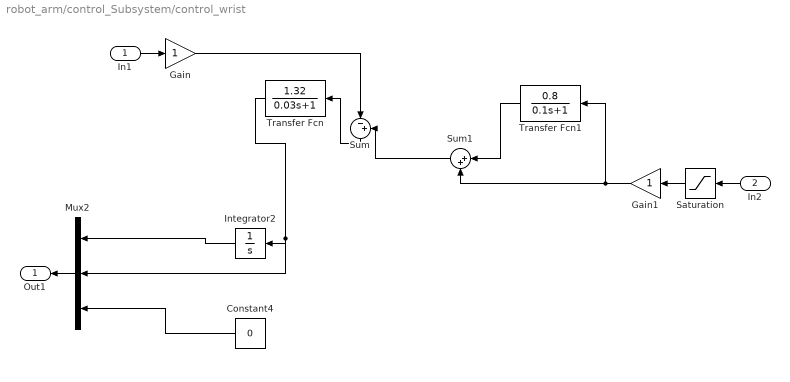
== system robot_arm/control_Subsystem/control_wrist ==
  In1 : Inport
  In2 : Inport  Orientation=left  Port=2
  Constant4 : Constant  Orientation=left  Value=0  OutDataType=sfix(16)  OutScaling=2^0
  Gain : Gain  ParameterDataType=sfix(16)  ParameterScaling=2^0  OutDataType=sfix(16)  OutScaling=2^0
  Gain1 : Gain  Orientation=left  ParameterDataType=sfix(16)  ParameterScaling=2^0  OutDataType=sfix(16)  OutScaling=2^0
  Integrator2 : Integrator  Orientation=left
  Mux2 : Mux  Orientation=left  Inputs=3
  Saturation : Saturate  Orientation=left  UpperLimit=80  LowerLimit=-90  OutMin=[-90]  OutMax=[90]  OutDataType=sfix(16)  OutScaling=2^0
  Sum : Sum  Orientation=down  Inputs=|-+  OutDataType=sfix(16)  OutScaling=2^0
  Sum1 : Sum  Orientation=left  Inputs=|++  OutDataType=sfix(16)  OutScaling=2^0
  Transfer Fcn : TransferFcn  Orientation=left  Numerator=[1.32]  Denominator=[0.03 1]
  Transfer Fcn1 : TransferFcn  Orientation=left  Numerator=[0.8]  Denominator=[0.1 1]
  Out1 : Outport  Orientation=left
  wires:
  Sum/1 -> Transfer Fcn/1
  Gain/1 -> Sum/1
  Integrator2/1 -> Mux2/1
  Transfer Fcn/1 -> Integrator2/1, Mux2/2
  Constant4/1 -> Mux2/3
  In1/1 -> Gain/1
  In2/1 -> Saturation/1
  Mux2/1 -> Out1/1
  Sum1/1 -> Sum/2
  Saturation/1 -> Gain1/1
  Gain1/1 -> Transfer Fcn1/1, Sum1/2
  Transfer Fcn1/1 -> Sum1/1
